simulink model "control"  (R2022b)
settings: Solver=VariableStepAuto  StartTime=0.0  StopTime=3.4  RelTol=1e-3
values from neighbouring files (symbols this model uses):
  q0 = [-0.927293431585 -1.28700579042 0.7 2.21429922201]    [generated_traj.mat]
  Ts = 0.001    [generated_traj.mat]
undefined symbols (not defined in the file or in its folder): DiscIntNeverNeededParam
settings Model: Creator=giuseppeloianno  LastModifiedBy=abidp
settings DataIOCC: ReturnWorkspaceOutputs=off

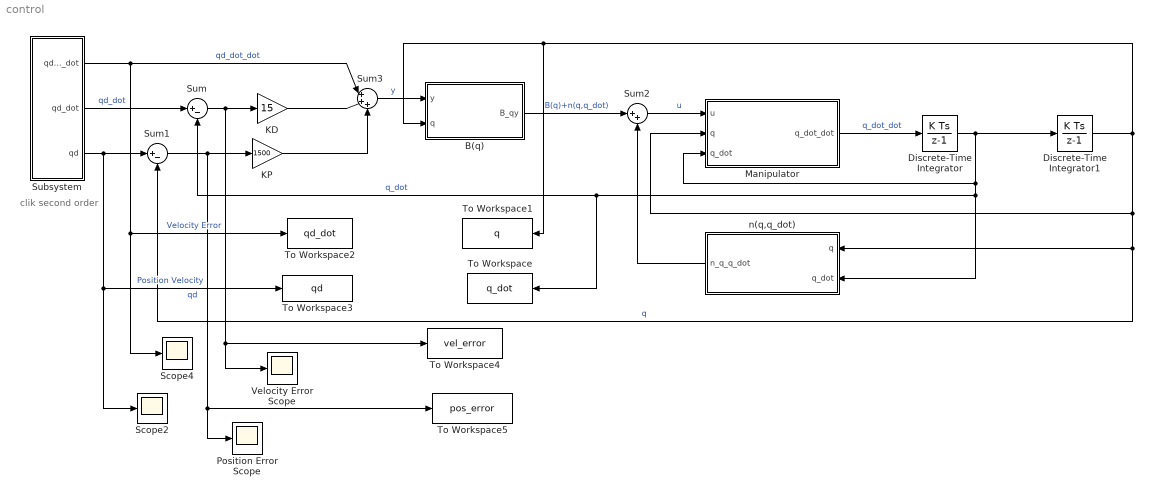
== system control ==
  note: clik second order
  B(q) : MATLAB Function  TreatAsAtomicUnit=on
  Discrete-Time Integrator : DiscreteIntegrator  InitialCondition=[0;0;0;0]  SampleTime=Ts  ICPrevOutput=DiscIntNeverNeededParam  ICPrevScaledInput=DiscIntNeverNeededParam
  Discrete-Time Integrator1 : DiscreteIntegrator  InitialCondition=q0  SampleTime=Ts  LimitOutput=on  UpperSaturationLimit=[pi/2;pi/4;1;2*pi]  LowerSaturationLimit=[-pi/2;-pi/2;0.25;-2*pi]  ICPrevOutput=DiscIntNeverNeededParam  ICPrevScaledInput=DiscIntNeverNeededParam
  KD : Gain  Gain=15
  KP : Gain  Gain=1500
  Manipulator : MATLAB Function  TreatAsAtomicUnit=on
  Position Error Scope : Scope
  Scope2 : Scope
  Scope4 : Scope
  Subsystem : Subsystem
  Sum : Sum  Inputs=|+-
  Sum1 : Sum  Inputs=|+-
  Sum2 : Sum  Inputs=|++
  Sum3 : Sum  Inputs=|+++
  To Workspace : ToWorkspace  VariableName=q_dot  SampleTime=-1
  To Workspace1 : ToWorkspace  VariableName=q  SampleTime=-1
  To Workspace2 : ToWorkspace  VariableName=qd_dot  SampleTime=-1
  To Workspace3 : ToWorkspace  VariableName=qd  SampleTime=-1
  To Workspace4 : ToWorkspace  VariableName=vel_error  SampleTime=-1
  To Workspace5 : ToWorkspace  VariableName=pos_error  SampleTime=-1
  Velocity Error Scope : Scope
  n(q,q_dot) : MATLAB Function  TreatAsAtomicUnit=on
  wires:
  B(q)/1(B_qy) -> Sum2/1  "B(q)+n(q,q_dot)"
  Sum2/1 -> Manipulator/1(u)  "u"
  n(q,q_dot)/1(n_q_q_dot) -> Sum2/2
  Sum3/1 -> B(q)/1(y)  "y"
  Manipulator/1(q_dot_dot) -> Discrete-Time Integrator/1  "q_dot_dot"
  Discrete-Time Integrator/1 -> Manipulator/3(q_dot), To Workspace/1, Sum/2, n(q,q_dot)/2(q_dot), Discrete-Time Integrator1/1  "q_dot"
  Discrete-Time Integrator1/1 -> To Workspace1/1, B(q)/2(q), Manipulator/2(q), n(q,q_dot)/1(q), Sum1/2  "q"
  Sum1/1 -> Position Error Scope/1, To Workspace5/1, KP/1  "Position Velocity"
  Sum/1 -> KD/1, Velocity Error Scope/1, To Workspace4/1  "Velocity Error"
  Subsystem/3(qd) -> To Workspace3/1, Scope2/1, Sum1/1  "qd"
  Subsystem/2(qd_dot) -> Sum/1  "qd_dot"
  KP/1 -> Sum3/3
  Subsystem/1(qd_dot_dot) -> To Workspace2/1, Scope4/1, Sum3/1  "qd_dot_dot"
  KD/1 -> Sum3/2

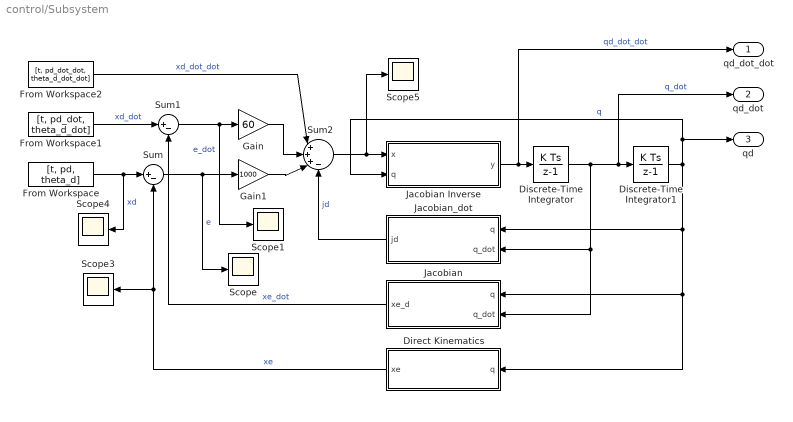
== system control/Subsystem ==
  Direct Kinematics : MATLAB Function  TreatAsAtomicUnit=on
  Discrete-Time Integrator : DiscreteIntegrator  InitialCondition=[0;0;0;0]  SampleTime=Ts  ICPrevOutput=DiscIntNeverNeededParam  ICPrevScaledInput=DiscIntNeverNeededParam
  Discrete-Time Integrator1 : DiscreteIntegrator  InitialCondition=q0  SampleTime=Ts  LimitOutput=on  UpperSaturationLimit=[pi/2;pi/4;1;2*pi]  LowerSaturationLimit=[-pi/2;-pi/2;0.25;-2*pi]  ICPrevOutput=DiscIntNeverNeededParam  ICPrevScaledInput=DiscIntNeverNeededParam
  From Workspace : FromWorkspace  VariableName=[t, pd, theta_d]  OutDataTypeStr=double  SampleTime=Ts
  From Workspace1 : FromWorkspace  VariableName=[t, pd_dot, theta_d_dot]  SampleTime=Ts
  From Workspace2 : FromWorkspace  VariableName=[t, pd_dot_dot, theta_d_dot_dot]  OutDataTypeStr=double  SampleTime=Ts
  Gain : Gain  Gain=60
  Gain1 : Gain  Gain=1000
  Jacobian : MATLAB Function  TreatAsAtomicUnit=on
  Jacobian Inverse : MATLAB Function  TreatAsAtomicUnit=on
  Jacobian_dot : MATLAB Function  TreatAsAtomicUnit=on
  Scope{,1,3..5} (5 alike) : Scope
  Sum : Sum  Inputs=|+-
  Sum1 : Sum  Inputs=|+-
  Sum2 : Sum  Inputs=|+++-
  qd_dot_dot : Outport
  qd_dot : Outport  Port=2
  qd : Outport  Port=3
  wires:
  Discrete-Time Integrator1/1 -> Jacobian Inverse/2(q), qd/1, Direct Kinematics/1(q), Jacobian/1(q), Jacobian_dot/1(q)  "q"
  Jacobian/1(xe_d) -> Sum1/2  "xe_dot"
  Jacobian Inverse/1(y) -> qd_dot_dot/1, Discrete-Time Integrator/1  "qd_dot_dot"
  Discrete-Time Integrator/1 -> qd_dot/1, Discrete-Time Integrator1/1, Jacobian/2(q_dot), Jacobian_dot/2(q_dot)  "q_dot"
  From Workspace/1 -> Scope4/1, Sum/1  "xd"
  Gain/1 -> Sum2/2
  Sum/1 -> Scope/1, Gain1/1  "e"
  Sum2/1 -> Scope5/1, Jacobian Inverse/1(x)
  Sum1/1 -> Scope1/1, Gain/1  "e_dot"
  Direct Kinematics/1(xe) -> Sum/2, Scope3/1  "xe"
  From Workspace1/1 -> Sum1/1  "xd_dot"
  Jacobian_dot/1(jd) -> Sum2/4  "jd"
  Gain1/1 -> Sum2/3
  From Workspace2/1 -> Sum2/1  "xd_dot_dot"

== matlab function control/Subsystem/Direct Kinematics ==
  data: q input; xe output
function xe = direct_kin(q)
    %xe = [0 0 0 0];
    xe = direct_kin(q);
end

== matlab function control/Subsystem/Jacobian_dot ==
  data: q input; jd output; q_dot input
function jd = jacobian_dot(q, q_dot)
    jd = jacobian_dot(q, q_dot);
end

== matlab function control/Subsystem/Jacobian Inverse ==
  data: x input; y output; q input
function y = jacobian_inverse(x,q)
    y = [0; 0; 0; 0;];
    y = jacobian_inverse(x,q);
end

== matlab function control/B(q) ==
  data: y input; B_qy output; q input
function B_qy = B(y,q)
    B_qy = B(y,q);
end

== matlab function control/Manipulator ==
  data: u input; q_dot_dot output; q input; q_dot input
function q_dot_dot = manipulator(u, q, q_dot)
    q_dot_dot = manipulator(u, q, q_dot);
end

== matlab function control/n(q,q_dot) ==
  data: q input; n_q_q_dot output; q_dot input
function n_q_q_dot = n(q, q_dot)
    n_q_q_dot = n(q, q_dot);
end

== matlab function control/Subsystem/Jacobian ==
  data: q input; xe_d output; q_dot input
function xe_d  = jacobian(q, q_dot)
    [~, xe_d] = jacobian(q, q_dot);
end
